simulink model "sistemaelectrico1"  (R2022b)
settings: Solver=VariableStepAuto  StartTime=0.0  StopTime=0.01  MaxStep=.0001  RelTol=1e-3
values from neighbouring files (symbols this model uses):
  c = .00001    (= 1e-05)    [ValoresInicialesCDCD.m]
  l = .002    (= 0.002)    [ValoresInicialesCDCD.m]
  r = 10    [ValoresInicialesCDCD.m]
  vin = 32    [ValoresInicialesCDCD.m]
libraries: simulink x1
settings Model: Creator=bryan  LastModifiedBy=perez

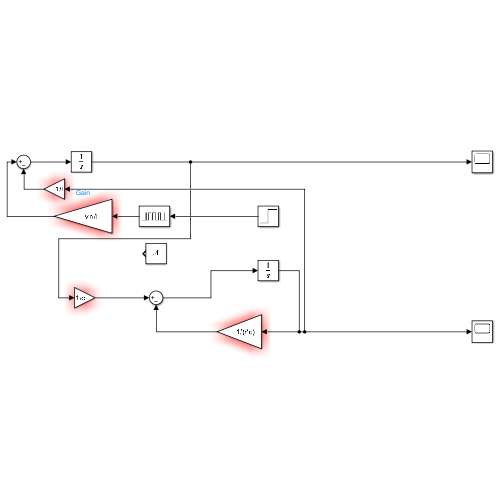
[thumbnail: Simulink's stored preview of the top-level diagram]
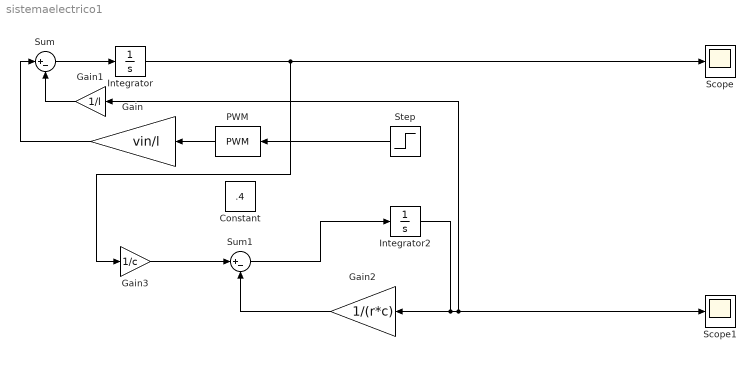
== system sistemaelectrico1 ==
  Constant : Constant  Value=.4
  Gain : Gain  Gain=vin/l
  Gain1 : Gain  Gain=1/l
  Gain2 : Gain  Gain=1/(r*c)
  Gain3 : Gain  Gain=1/c
  Integrator : Integrator
  Integrator2 : Integrator
  PWM : simulink/Discontinuities/PWM  DisableCoverage=on  Period=1/100000  InitialDelay=0  DisallowZeroDutyCycle=off  RunAtFixedTimeIntervals=on  SampleTime=1/1000000
  Scope : Scope
  Scope1 : Scope
  Step : Step  Before=.4  SampleTime=0
  Sum : Sum  Inputs=|+-
  Sum1 : Sum  Inputs=|+-
  wires:
  Integrator/1 -> Scope/1, Gain3/1
  Integrator2/1 -> Gain2/1, Scope1/1, Gain1/1
  Sum/1 -> Integrator/1
  Sum1/1 -> Integrator2/1
  Gain1/1 -> Sum/2
  Gain/1 -> Sum/1
  Gain2/1 -> Sum1/2
  Gain3/1 -> Sum1/1
  Step/1 -> PWM/1
  PWM/1 -> Gain/1
